simulink model "Simulink_Sim_Plant"  (R2024b)
settings: Solver=VariableStepAuto  StartTime=0.0  StopTime=10  RelTol=1e-3
values from neighbouring files (symbols this model uses):
  Ts = para1.looptime * 1.0e-6    [Plots_doku_angle.m]    (also in Plots_doku_gyro.m; Simulation.m = para.looptime * 1.0e-6; Simulation_Plant.m = 0.000125; Simulation_Regler.m = para.looptime * 1.0e-6)
libraries: cstblocks x1
settings Model: Creator=janic  LastModifiedBy=janic

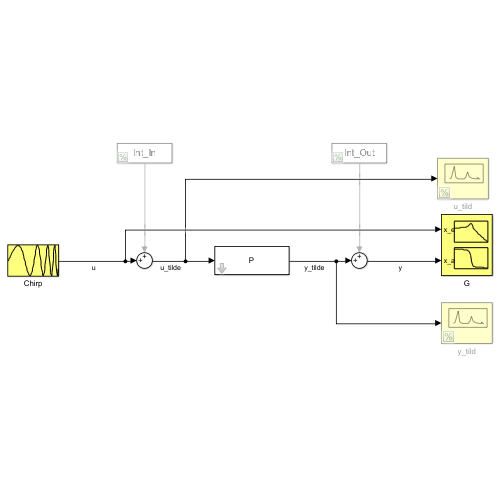
[thumbnail: Simulink's stored preview of the top-level diagram]
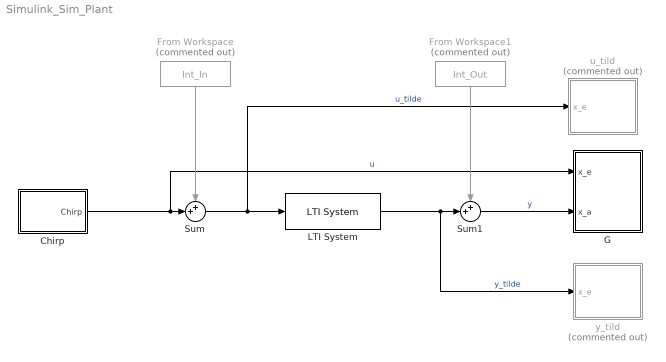
== system Simulink_Sim_Plant ==
  Chirp : Subsystem  LoadFcn=|  mask(bode_chirp){mode=logarithmic, f1=0.1, f2=4000, ampl=1, offs=0, T0=0, Tm=10, editSweepTime=off, Trig=1, mode_n=2, Dummy=0}
      | try
      |  ZHAWcbfcn('defaultchirp');
      | end
      mask prompts: mode "Sweep Sine Mode"; f1 "Start Frequency [Hz]"; f2 "End Frequency [Hz]"; ampl "Amplitude"; offs "Offset"; T0 "Settle Time [s]"; Tm "Sweep Time [s]"; editSweepTime "Edit"; Trig "Trigger"; mode_n "Chirp Mode"
      mask help: Creates a chirp (sweep sinus) signal used for gain phase analyzer.
      settings: OpenFcn=try ZHAWcbfcn('openMask'); end
      settings: CopyFcn=|
      | set_param(gcb,'LinkStatus',getpref('ZHAW_SLDRT_lib','LibraryLinkStatus','none'));
      | try
      |  set_param(gcb,'f2',num2str(1/evalin('base','Ts')/2))
      | end
      | try
      |  ZHAWcbfcn('SimTime');
      | end
      | try
      |  ZHAWcbfcn('defaultchirp');
      | end
      | set_param(gcb,'OpenFcn','try ZHAWcbfcn(''openMask''); end')
      mask TypeOptions mode: linear | logarithmic | quadratic
      mask Callback mode:
      | try
      | ZHAWcbfcn('ChirpMode')
      | end
      mask Callback f1:
      | try
      |     ZHAWcbfcn('fstart')
      | end
      | try
      |     ZHAWcbfcn('SimTime')
      | end
      | try
      |     ZHAWcbfcn('editSweepTime')
      | end
      mask Callback f2:
      | try
      |     ZHAWcbfcn('fend')
      | end
      mask Callback ampl:
      | try
      | ZHAWcbfcn('ApplyChanges')
      | end
      mask Callback offs:
      | try
      | ZHAWcbfcn('ApplyChanges')
      | end
      mask Callback T0:
      | try
      |     ZHAWcbfcn('SettleTime')
      | end
      | try
      |     ZHAWcbfcn('SimTime')
      | end
      mask Callback Tm:
      | try
      | ZHAWcbfcn('SimTime')
      | end
      mask Callback editSweepTime:
      | try
      | ZHAWcbfcn('editSweepTime')
      | end
      | try
      | ZHAWcbfcn('SimTime')
      | end
      mask DialogControl DescGroupVar Prompt: Chirp Signal Generator (R2024a)
      mask DialogControl Control3 Prompt: Manuel Trigger Chirp
      mask DialogControl Control3 Callback:
      | try
      |     ZHAWcbfcn('TrigChirpClb')
      | end
      mask Display: plot(chirp(0:0.1:10,0.1,10,1,'logarithmic',-90))
  From Workspace : FromWorkspace  Commented=on  VariableName=Int_In
  From Workspace1 : FromWorkspace  Commented=on  VariableName=Int_Out  SampleTime=Ts  OutputAfterFinalValue=Setting to zero
  G : Subsystem  LoadFcn=|  StopFcn=|  mask(gpa){funits=Hz, aunits=dB, punits=deg, fstart=0.1, edit_fstart=off, fend=4000, edit_fend=off, unwrap=wrap phase +/-180°, integ=off, shiftphase=0, Tsettle=0, editTsettle=off, Wlen=, wintyp=hann, fig=gcf, hmode=off, coherence=off, auto_gpa=on}
      | try
      |  ZHAWcbfcn('default');
      | end
      | try
      |  ZHAWcbfcn('bode');
      | end
      mask prompts: funits "Frequency Units"; aunits "Amplitude Units"; punits "Phase Units"; fstart "Minimum Frequency [Hz]:"; edit_fstart "Edit"; fend "Maximum Frequency [Hz]:"; edit_fend "Edit"; unwrap "Unwrap Phase"; integ "System has integral behavior"; shiftphase "Delay-Time for Phase Shift [s]:"; Tsettle "Truncate Settle Time [s]:"; editTsettle "Edit"; Wlen "Window Length:"; wintyp "Window:"; fig "Figure:"; hmode "Hold Current Axes"; coherence "Plot Coherence"; auto_gpa "Calc Bode after Simulation Stop"
      mask help:
      | Calculate and plot bode diagram using tfestimate.
      | The block name is used to create an FRD-object in the workspace.
      | Default window length (empty) does split the FRF in several sections with optimized averaging.
      mask init:
      | blk = gcb;
      | ind = strfind(blk,'/');
      | data = [blk(ind(end)+1:end),'_td'];
      | set_param([blk,'/To Workspace'],'VariableName',data)
      | try
      |     ZHAWcbfcn('bodeoptions')
      | end
      settings: NameChangeFcn=try ZHAWcbfcn('namechangeGPA'); end  OpenFcn=try ZHAWcbfcn('openMask'); end
      settings: CopyFcn=|
      | try
      | ZHAWcbfcn('copyGPA');
      | end
      | set_param(gcb,'OpenFcn','try ZHAWcbfcn(''openMask''); end')
      mask Help:
      | Window length:
      |     empty:
      |         first section with no averages (window length=#sample) (no window)
      |         second section with 10 averages (window as specified)
      |         third section with 100 averages (window as specified)
      |         ...
      | inf:
      |     no averages (window length=#sample) (window as specified)
      | 
      | overlap: 50%
      mask TypeOptions funits: Hz | rad/s
      mask Callback funits:
      | try
      |     ZHAWcbfcn('bodeoptions')
      | end
      mask TypeOptions aunits: dB | abs
      mask Callback aunits:
      | try
      |     ZHAWcbfcn('bodeoptions')
      | end
      mask TypeOptions punits: rad | deg
      mask Callback punits:
      | try
      |     ZHAWcbfcn('bodeoptions')
      | end
      mask Callback fstart:
      | try
      |     ZHAWcbfcn('gpafstart')
      | end
      | try
      |     ZHAWcbfcn('bodeoptions')
      | end
      mask Callback edit_fstart:
      | try
      |     ZHAWcbfcn('edit_fstart');
      | end
      | try
      |     ZHAWcbfcn('fstart');
      | end
      mask Callback fend:
      | try
      |     ZHAWcbfcn('gpafend')
      | end
      | try
      |     ZHAWcbfcn('bodeoptions')
      | end
      mask Callback edit_fend:
      | try
      |     ZHAWcbfcn('edit_fend');
      | end
      | try
      |     ZHAWcbfcn('fend');
      | end
      mask TypeOptions unwrap: wrap phase +/-180° | unwrap phase
      mask Callback unwrap:
      | try
      |     ZHAWcbfcn('bodeoptions')
      | end
      mask Callback editTsettle:
      | try
      |     ZHAWcbfcn('editTsettle')
      | end
      | try
      |     ZHAWcbfcn('SettleTime')
      | end
      mask TypeOptions wintyp: barthannwin | bartlett | blackman | blackmanharris | bohmanwin | chebwin | flattopwin | gausswin | hamming | hann | kaiser | nuttallwin | parzenwin | rectwin | taylorwin | triang | tukeywin
      mask DialogControl DescGroupVar Prompt: Gain Phase Analyzer (R2024a)
      mask DialogControl Control2 Prompt: help tfetimate
      mask DialogControl Control2 Callback: doc tfestimate
      mask DialogControl Container4 Prompt: Basic
      mask DialogControl Container5 Prompt: Advanced (changes need to recalc bode)
      mask DialogControl Control3 Prompt: Calc Bode Manually
      mask DialogControl Control3 Callback:
      | try
      |     ZHAWcbfcn('bode',1);
      | end
      mask Display:
      | mat = [
      |    10.0000   78.3832   42.8007
      |    11.6327   78.3936   42.7806
      |    13.2653   78.4061   42.7584
      |    14.8980   78.4213   42.7338
      |    16.5306   78.4397   42.7064
      |    18.1633   78.4620   42.6761
      |    19.7959   78.4890   42.6423
      |    21.4286   78.5217   42.6044
      |    23.0612   78.5616   42.5620
      |    24.6939   78.6100   42.5142
      |    26.3265   78.6691   42.4600
      |    27.9592   78.7412   42.3982
      |    29.5918   78.8296   42.3272
      |    31.2245   78.9383   42.2447
      |    32.8571   79.0724   42.1478
      |    34.4898   79.2389   42.0322
      |    36.1224   79.4469   41.8917
      |    37.7551   79.7090   41.7169
      |    39.3878   80.0430   41.4928
      |    41.0204   80.4749   41.1939
      |    42.6531   81.0442   40.7735
      |    44.2857   81.8142   40.1368
      |    45.9184   82.8890   39.0620
      |    47.5510   84.4186   36.9274
      |    49.1837   86.2203   31.8362
      |    50.8163   85.7441   23.1638
      |    52.4490   82.9900   18.0726
      |    54.0816   80.5081   15.9380
      |    55.7143   78.4809   14.8632
      |    57.3469   76.7585   14.2265
      |    58.9796   75.2368   13.8061
      |    60.6122   73.8525   13.5072
      |    62.2449   72.5661   13.2831
      |    63.8776   71.3516   13.1083
      |    65.5102   70.1913   12.9678
      |    67.1429   69.0724   12.8522
      |    68.7755   67.9859   12.7553
      |    70.4082   66.9248   12.6728
      |    72.0408   65.8841   12.6018
      |    73.6735   64.8595   12.5400
      |    75.3061   63.8481   12.4858
      |    76.9388   62.8473   12.4380
      |    78.5714   61.8551   12.3956
      |    80.2041   60.8699   12.3577
      |    81.8367   59.8905   12.3239
      |    83.4694   58.9159   12.2936
      |    85.1020   57.9451   12.2662
      |    86.7347   56.9776   12.2416
      |    88.3673   56.0126   12.2194
      |    90.0000   55.0499   12.1993
      | ];
      | plot(-20,0,...
      |     100,100,...
      |     [10,90,90,10,10], [45,45,10,10,45],...
      |     [10,90,90,10,10], [90,90,55,55,90],...
      |     mat(:,1),mat(:,2),mat(:,1),mat(:,3));
  LTI System : cstblocks/LTI System  sys=P  IC=[]  PadeOrder=0
  Sum : Sum  Inputs=++|
  Sum1 : Sum  Inputs=++|
  u_tild : Subsystem  Commented=on  StopFcn=|  mask(Spectrum Plot){funits=Hz, aunits=dB, punits=deg, amp=on, phase=off, wintyp=rectwin, flog=on, fig=gcf, hold_mode=off}
      | try
      |  ZHAWcbfcn('Spec');
      | end
      mask prompts: funits "Frequency Units"; aunits "Amplitude Units"; punits "Phase Units"; amp "Show Amplitude Spectrum"; phase "Show Phase Spectrum"; wintyp "Window:"; flog "Logarithmic Frequency Scale"; fig "Figure:"; hold_mode "Hold Current Axis"
      mask help:
      | Plot spectrum of input signal.
      | Time data will be saved in workspace.
      mask init:
      | blk = gcb;
      | ind = strfind(blk,'/');
      | data = [blk(ind(end)+1:end),'_td'];
      | set_param([blk,'/To Workspace'],'VariableName',data)
      settings: NameChangeFcn=try ZHAWcbfcn('namechangeGPA'); end  OpenFcn=try ZHAWcbfcn('openMask'); end
      settings: CopyFcn=|
      | try
      | ZHAWcbfcn('copySPEC');
      | end
      | set_param(gcb,'OpenFcn','try ZHAWcbfcn(''openMask''); end')
      mask TypeOptions funits: Hz | rad/s
      mask TypeOptions aunits: linear | dB
      mask TypeOptions punits: deg | rad
      mask TypeOptions wintyp: barthannwin | bartlett | blackman | blackmanharris | bohmanwin | chebwin | flattopwin | gausswin | hamming | hann | kaiser | nuttallwin | parzenwin | rectwin | taylorwin | triang | tukeywin
      mask DialogControl DescGroupVar Prompt: Spectrum Plot (R2024a)
      mask DialogControl ParameterTabVar0 Prompt: Basic
      mask DialogControl Container4 Prompt: Advanced
      mask DialogControl Control2 Prompt: Plot Spectrum
      mask DialogControl Control2 Callback:
      | try
      |     ZHAWcbfcn('Spec');
      | end
      mask Display: plot(0,0,100,100,[14,91,91,14,14],[86,86,40,40,86],[85,82,80,79,75,67,63,60,57,53,41,36,33,27,24],[49,50,53,50,49,51,54,66,54,50,50,52,81,51,49])
  y_tild : Subsystem  Commented=on  StopFcn=|  mask(Spectrum Plot){funits=Hz, aunits=dB, punits=deg, amp=on, phase=off, wintyp=rectwin, flog=on, fig=gcf, hold_mode=off}
      | try
      |  ZHAWcbfcn('Spec');
      | end
      mask prompts: funits "Frequency Units"; aunits "Amplitude Units"; punits "Phase Units"; amp "Show Amplitude Spectrum"; phase "Show Phase Spectrum"; wintyp "Window:"; flog "Logarithmic Frequency Scale"; fig "Figure:"; hold_mode "Hold Current Axis"
      mask help:
      | Plot spectrum of input signal.
      | Time data will be saved in workspace.
      mask init:
      | blk = gcb;
      | ind = strfind(blk,'/');
      | data = [blk(ind(end)+1:end),'_td'];
      | set_param([blk,'/To Workspace'],'VariableName',data)
      settings: NameChangeFcn=try ZHAWcbfcn('namechangeGPA'); end  OpenFcn=try ZHAWcbfcn('openMask'); end
      settings: CopyFcn=|
      | try
      | ZHAWcbfcn('copySPEC');
      | end
      | set_param(gcb,'OpenFcn','try ZHAWcbfcn(''openMask''); end')
      mask TypeOptions funits: Hz | rad/s
      mask TypeOptions aunits: linear | dB
      mask TypeOptions punits: deg | rad
      mask TypeOptions wintyp: barthannwin | bartlett | blackman | blackmanharris | bohmanwin | chebwin | flattopwin | gausswin | hamming | hann | kaiser | nuttallwin | parzenwin | rectwin | taylorwin | triang | tukeywin
      mask DialogControl DescGroupVar Prompt: Spectrum Plot (R2024a)
      mask DialogControl ParameterTabVar0 Prompt: Basic
      mask DialogControl Container4 Prompt: Advanced
      mask DialogControl Control2 Prompt: Plot Spectrum
      mask DialogControl Control2 Callback:
      | try
      |     ZHAWcbfcn('Spec');
      | end
      mask Display: plot(0,0,100,100,[14,91,91,14,14],[86,86,40,40,86],[85,82,80,79,75,67,63,60,57,53,41,36,33,27,24],[49,50,53,50,49,51,54,66,54,50,50,52,81,51,49])
  wires:
  Chirp/1(Chirp) -> G/1(x_e), Sum/2  "u"
  Sum/1 -> u_tild/1(x_e), LTI System/1  "u_tilde"
  LTI System/1 -> y_tild/1(x_e), Sum1/2  "y_tilde"
  Sum1/1 -> G/2(x_a)  "y"
  From Workspace/1 -> Sum/1
  From Workspace1/1 -> Sum1/1

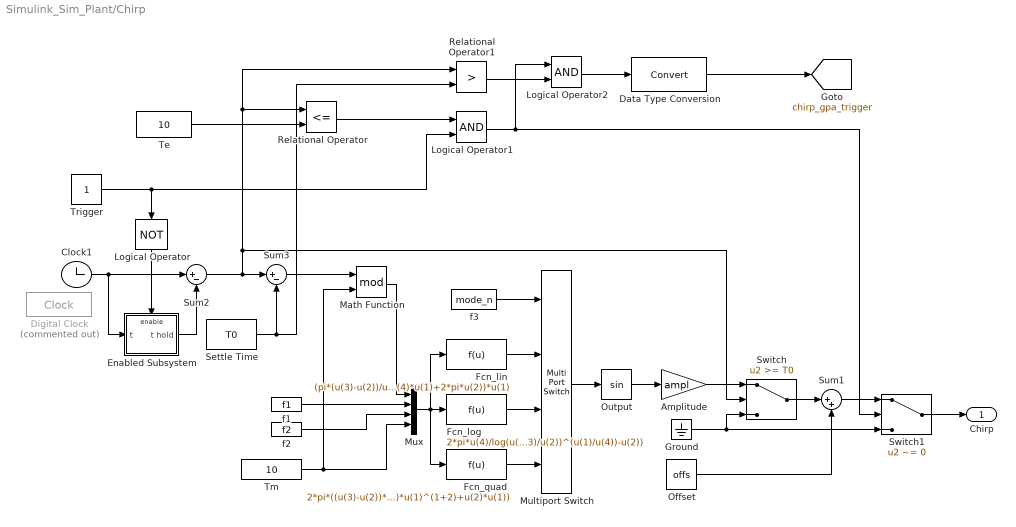
== system Simulink_Sim_Plant/Chirp ==
  Amplitude : Gain  Gain=ampl
  Clock1 : Clock
      settings: DisableCoverage=on
  Data Type Conversion : DataTypeConversion  SaturateOnIntegerOverflow=off  RndMeth=Floor
  Digital Clock : DigitalClock  Commented=on  SampleTime=Ts
  Enabled Subsystem : Subsystem  TreatAsAtomicUnit=on
  Fcn_lin : Fcn  Expr=(pi*(u(3)-u(2))/u(4)*u(1)+2*pi*u(2))*u(1)
  Fcn_log : Fcn  Expr=2*pi*u(4)/log(u(3)/u(2))*(u(2)*(u(3)/u(2))^(u(1)/u(4))-u(2))
  Fcn_quad : Fcn  Expr=2*pi*((u(3)-u(2))*u(4)^(-2)/(1+2)*u(1)^(1+2)+u(2)*u(1))
  Ground : Ground
  Logical Operator : Logic  Operator=NOT  AllPortsSameDT=off  OutDataTypeStr=boolean
  Logical Operator1 : Logic  AllPortsSameDT=off
  Logical Operator2 : Logic  AllPortsSameDT=off
  Math Function : Math  Operator=mod  SignedPower=on
  Multiport Switch : MultiPortSwitch  SaturateOnIntegerOverflow=off  InputSameDT=off
  Mux : Mux
  Offset : Constant  Value=offs
  Output : Trigonometry
  Relational Operator : RelationalOperator  Operator=<=  RndMeth=Simplest  InputSameDT=off
  Relational Operator1 : RelationalOperator  Operator=>  RndMeth=Simplest  InputSameDT=off
  Settle Time : Constant  Value=T0
  Sum1 : Sum  Inputs=|++
  Sum2 : Sum  Inputs=|+-
  Sum3 : Sum  Inputs=|+-
  Switch : Switch  Threshold=T0  SaturateOnIntegerOverflow=off  InputSameDT=off
  Switch1 : Switch  Criteria=u2 ~= 0  SaturateOnIntegerOverflow=off  InputSameDT=off
  Te : Constant  Value=10
  Tm : Constant  Value=10
  Trigger : Constant
  f1 : Constant  Value=f1
  f2 : Constant  Value=f2
  f3 : Constant  Value=mode_n
  Chirp : Outport  VectorParamsAs1DForOutWhenUnconnected=off
  tag scope: chirp_gpa_trigger=global
  wires:
  Te/1 -> Relational Operator/2
  Logical Operator/1 -> Enabled Subsystem/Enable
  Enabled Subsystem/1(t hold) -> Sum2/2
  Trigger/1 -> Logical Operator1/2, Logical Operator/1
  f3/1 -> Multiport Switch/1
  Fcn_lin/1 -> Multiport Switch/2
  Fcn_log/1 -> Multiport Switch/3
  Fcn_quad/1 -> Multiport Switch/4
  Multiport Switch/1 -> Output/1
  Math Function/1 -> Mux/1
  f2/1 -> Mux/3
  f1/1 -> Mux/2
  Mux/1 -> Fcn_log/1, Fcn_lin/1, Fcn_quad/1
  Clock1/1 -> Enabled Subsystem/1(t), Sum2/1
  Output/1 -> Amplitude/1
  Offset/1 -> Sum1/2
  Sum3/1 -> Math Function/1
  Tm/1 -> Mux/4, Math Function/2
  Switch/1 -> Sum1/1
  Amplitude/1 -> Switch/1
  Ground/1 -> Switch1/3, Switch/3
  Settle Time/1 -> Relational Operator1/2, Sum3/2
  Sum2/1 -> Switch/2, Relational Operator1/1, Relational Operator/1, Sum3/1
  Switch1/1 -> Chirp/1
  Sum1/1 -> Switch1/1
  Relational Operator/1 -> Logical Operator1/1
  Logical Operator1/1 -> Logical Operator2/1, Switch1/2
  Logical Operator2/1 -> Data Type Conversion/1
  Data Type Conversion/1 -> [chirp_gpa_trigger]
  Relational Operator1/1 -> Logical Operator2/2

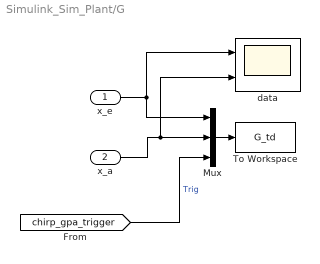
== system Simulink_Sim_Plant/G ==
  x_e : Inport
  x_a : Inport  Port=2
  Mux : Mux  Inputs=3
  To Workspace : ToWorkspace  VariableName=G_td  SaveFormat=Structure With Time  SampleTime=Ts
  data : Scope  NumInputPorts=2
      settings: CopyFcn=try ZHAWcbfcn('copyScope'); end  NameChangeFcn=try ZHAWcbfcn('namechangeScope'); end
  wires:
  x_e/1 -> data/1, Mux/1
  x_a/1 -> data/2, Mux/2
  Mux/1 -> To Workspace/1
  [chirp_gpa_trigger] -> Mux/3  "Trig"

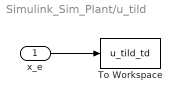
== system Simulink_Sim_Plant/u_tild ==
  x_e : Inport
  To Workspace : ToWorkspace  VariableName=u_tild_td  SaveFormat=Structure With Time  SampleTime=Ts
  wires:
  x_e/1 -> To Workspace/1

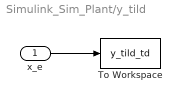
== system Simulink_Sim_Plant/y_tild ==
  x_e : Inport
  To Workspace : ToWorkspace  VariableName=y_tild_td  SaveFormat=Structure With Time  SampleTime=Ts
  wires:
  x_e/1 -> To Workspace/1

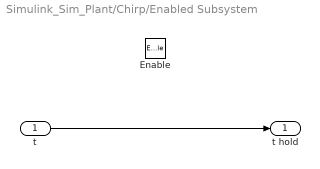
== system Simulink_Sim_Plant/Chirp/Enabled Subsystem ==
  t : Inport
  Enable : EnablePort
  t hold : Outport  VectorParamsAs1DForOutWhenUnconnected=off
  wires:
  t/1 -> t hold/1
